simulink model "simulazione_002_s"  (R2016b)
settings: Solver=ode4  StartTime=0.0  StopTime=t_sim  FixedStep=step  RelTol=1e-3
values from neighbouring files (symbols this model uses):
  gain = 30 * eye(6)    [simulazione_002_init.m]
  motion_time = 4    [simulazione_002_init.m]
  movement_lower_limit = -movement_upper_limit    [simulazione_002_init.m]
  movement_upper_limit = [2*pi; 2*pi; 2*pi; 2*pi; 2*pi; 2*pi]    [simulazione_002_init.m]
  p_init = direct_kinematic(q_init)    [simulazione_002_init.m]
  q_init = [0; 0; 0; -pi/2; 0; 0]    [simulazione_002_init.m]
  radius = 0.3    [simulazione_002_init.m]
  ref_pulse = 2 * pi * frequency    (= 3.14159265359)    [simulazione_002_init.m]
  velocity_lower_limit = -velocity_upper_limit    [simulazione_002_init.m]
  velocity_upper_limit = [2*pi/3; 2*pi/3; pi; pi; pi; pi]    [simulazione_002_init.m]
settings Model: Creator=IBM  LastModifiedBy=IBM

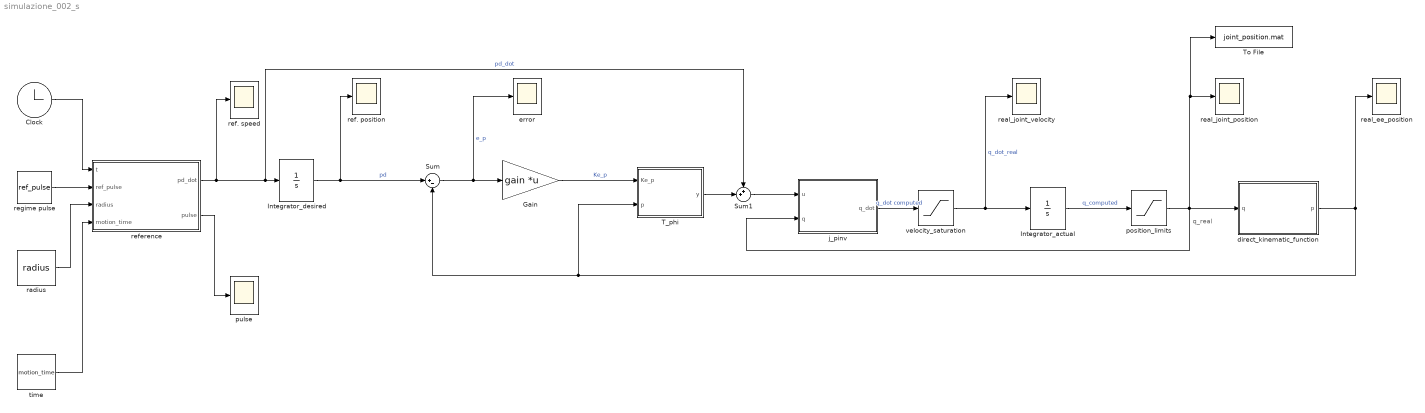
== system simulazione_002_s ==
  note: q_real
  Clock : Clock
  Gain : Gain  Gain=gain  Multiplication=Matrix(K*u) (u vector)
  Integrator_actual : Integrator  InitialCondition=q_init
  Integrator_desired : Integrator  InitialCondition=p_init
  Sum : Sum  Inputs=|+-
  Sum1 : Sum  Inputs=++|
  T_phi : MATLAB Function  TreatAsAtomicUnit=on
  To File : ToFile  Filename=joint_position.mat  MatrixName=q
  direct_kinematic_function : MATLAB Function  TreatAsAtomicUnit=on
  error : Scope
  j_pinv : MATLAB Function  TreatAsAtomicUnit=on
  position_limits : Saturate  UpperLimit=movement_upper_limit  LowerLimit=movement_lower_limit
  pulse : Scope
  radius : Constant  Value=radius
  real_ee_position : Scope
  real_joint_position : Scope
  real_joint_velocity : Scope
  ref. position : Scope
  ref. speed : Scope
  reference : MATLAB Function  TreatAsAtomicUnit=on
  regime pulse : Constant  Value=ref_pulse
  time : Constant  Value=motion_time
  velocity_saturation : Saturate  UpperLimit=velocity_upper_limit  LowerLimit=velocity_lower_limit
  wires:
  Clock/1 -> reference/1(t)
  Integrator_desired/1 -> ref. position/1, Sum/1  "pd"
  radius/1 -> reference/3(radius)
  Sum/1 -> error/1, Gain/1  "e_p"
  T_phi/1(y) -> Sum1/2
  Sum1/1 -> j_pinv/1(u)
  Integrator_actual/1 -> position_limits/1  "q_computed"
  direct_kinematic_function/1(p) -> real_ee_position/1, Sum/2, T_phi/2(p)
  regime pulse/1 -> reference/2(ref_pulse)
  reference/1(pd_dot) -> ref. speed/1, Sum1/1, Integrator_desired/1  "pd_dot"
  Gain/1 -> T_phi/1(Ke_p)  "Ke_p"
  time/1 -> reference/4(motion_time)
  reference/2(pulse) -> pulse/1
  j_pinv/1(q_dot) -> velocity_saturation/1  "q_dot computed"
  velocity_saturation/1 -> real_joint_velocity/1, Integrator_actual/1  "q_dot_real"
  position_limits/1 -> j_pinv/2(q), To File/1, real_joint_position/1, direct_kinematic_function/1(q)

== matlab function simulazione_002_s/j_pinv ==
  data: u input; q_dot output; q input
function q_dot = j_pinv(u, q)
    
    J = geometric_jacobian(q);
    J_p = pinv(J);
    q_dot = J_p*u;
    
end

== matlab function simulazione_002_s/reference ==
  data: t input; ref_pulse input; pd_dot output; radius input; motion_time input; pulse output
function [pd_dot, pulse] = reference(t, ref_pulse, radius, motion_time)

    [pd_dot, pulse] = circular_reference(t, ref_pulse, radius, motion_time);
    
end

== matlab function simulazione_002_s/direct_kinematic_function ==
  data: q input; p output
function p = dkf(q)

    p = direct_kinematic(q);

== matlab function simulazione_002_s/T_phi ==
  data: Ke_p input; y output; p input
function y = T_phi(Ke_p, p)
        
    t_phi_matrix = [0,  -sin(p(4)),     cos(p(4))*sin(p(5));
                    0,   cos(p(4)),     sin(p(4))*sin(p(5));
                    1,       0,             cos(p(5))];
            
    t_phi_matrix_6x6 = [ eye(3),   zeros(3);
                        zeros(3), t_phi_matrix];
    
    y = t_phi_matrix_6x6 * Ke_p;
end
